simulink model "planar_vtol_sim_2"  (R2018a)
settings: Solver=ode45  StartTime=0.0  StopTime=10000  RelTol=1e-3
InitFcn:
  | planar_vtol_param
undefined symbols (not defined in the file or in its folder): planar_vtol_animation
settings Model: Creator=canla  LastModifiedBy=canla
settings OptimizationCC: LifeSpan=inf

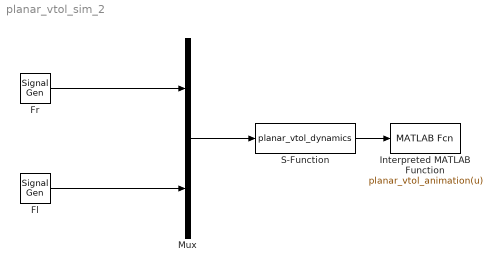
== system planar_vtol_sim_2 ==
  Fl : SignalGenerator  Amplitude=50  Frequency=10  Units=rad/sec
  Fr : SignalGenerator  Amplitude=50  Frequency=5  Units=rad/sec
  Interpreted MATLAB Function : MATLABFcn  MATLABFcn=planar_vtol_animation(u)  OutputDimensions=-0
  Mux : Mux  Inputs=2
  S-Function : S-Function  FunctionName=planar_vtol_dynamics  Parameters=P  SFunctionDeploymentMode=off  EnableBusSupport=off
  wires:
  Mux/1 -> S-Function/1
  S-Function/1 -> Interpreted MATLAB Function/1
  Fr/1 -> Mux/1
  Fl/1 -> Mux/2
